simulink model "UAV"  (R2024a)
settings: Solver=FixedStepAuto  StartTime=0  StopTime=inf  MaxStep=0.01  RelTol=1e-4
values from neighbouring files (symbols this model uses):
  actuatorCentres = 0.0    [data.sldd]
  datcom1 : value not decoded    [data.sldd]
  deflectionLimits = -10.0    [data.sldd]
  loggingSampleTime = 1.0    [data.sldd]
  sensorSampleTime = 0.02    [data.sldd]
  vehicle = 1.23    [data.sldd]
undefined symbols (not defined in the file or in its folder): aeroCoeff, aMode, DiscIntNeverNeededParam, Discrete, Earth, HDBK, MIL, Newton, pa28, Raphson, Time, WGS84
libraries: slpidlib x20, simulink_extras x15, simulink x13, arduinolib x8, aerolibasang x5, aerolibactuator x4, aerolibutil x4, aerolibtransform2 x4, sharedtransform x3, ctrlSharedLib x3, aerolibadyn x3, dspstat3 x2
(part 2 of 5)

== system UAV/Arduino/Actuators/Real Actuators/Initialize Function ==
  Aileron Servos : arduinolib/Standard Servo Write  pinNumber=servoPins.aileron.right  ServoIndex=0  blockPlatform=ARDUINO
  Elevator Servo : arduinolib/Standard Servo Write  pinNumber=servoPins.elevator.right  ServoIndex=0  blockPlatform=ARDUINO
  Event Listener : EventListener  DisableCoverage=on  EventName=reset
  Flap Servo : arduinolib/Standard Servo Write  pinNumber=servoPins.flap.right  ServoIndex=0  blockPlatform=ARDUINO
  Rudder Servo : arduinolib/Standard Servo Write  pinNumber=servoPins.rudder  ServoIndex=0  blockPlatform=ARDUINO
  Step : Step  After=180  SampleTime=0
  Step1 : Step  Time=6  After=180  SampleTime=0
  Sum : Sum  Inputs=+-
  wires:
  Sum/1 -> Flap Servo/1, Rudder Servo/1, Elevator Servo/1, Aileron Servos/1
  Step/1 -> Sum/1
  Step1/1 -> Sum/2

== system UAV/Arduino/Flight Control/Model Flight Control/Guidance States/Guidance.ALT_Hold.ALT ==
  Sensors : Inport  OutDataTypeStr=Bus: Sensors
  Demands : Inport  Port=2  OutDataTypeStr=Bus: Demands
  Control Override : Inport  Port=3  OutDataTypeStr=Bus: ControlOverrides
  Action Port : ActionPort
      settings: CopyFcn=Stateflow.SLINSF.SimulinkMan.removeBlockPreDeleteFcn  PreDeleteFcn=Stateflow.SLINSF.SimulinkMan.unsafePredeleteFcn
  Altitude Hold : Subsystem
  Bus Selector : BusSelector  OutputSignals=X_e,phi_theta_psi
  Bus Selector1 : BusSelector  OutputSignals=Altitude
  Bus Selector2 : BusSelector  OutputSignals=Aileron
  Mux : Mux  Inputs=2
  Radians to Degrees : simulink_extras/Transformations/Radians to Degrees
  Rate Limiter : RateLimiter  SampleTimeMode=inherited
  Selector1 : Selector  IndexMode=Zero-based  InputPortWidth=3  IndexOptions=Index vector (dialog)  Indices=[2]  OutputSizes=1
  Selector2 : Selector  IndexMode=Zero-based  InputPortWidth=3  IndexOptions=Index vector (dialog)  Indices=[1]  OutputSizes=1
  Commands : Outport  OutDataTypeStr=single  PortDimensions=2  SampleTime=sensorSampleTime  VectorParamsAs1DForOutWhenUnconnected=off
  wires:
  Mux/1 -> Commands/1
  Altitude Hold/1(Elevator) -> Mux/2
  Selector2/1 -> Radians to Degrees/1
  Sensors/1 -> Bus Selector/1
  Demands/1 -> Bus Selector1/1
  Bus Selector/1 -> Selector1/1  "<X_e>"
  Bus Selector/2 -> Selector2/1  "<phi_theta_psi>"
  Bus Selector1/1 -> Rate Limiter/1  "<Altitude>"
  Rate Limiter/1 -> Altitude Hold/2(Demanded ALT)
  Bus Selector2/1 -> Mux/1  "<Aileron>"
  Control Override/1 -> Bus Selector2/1
  Selector1/1 -> Altitude Hold/1(ALT)
  Radians to Degrees/1 -> Altitude Hold/3(theta)

== system UAV/Arduino/Flight Control/Model Flight Control/Guidance States/Guidance.HDG_ALT_Hold.HDG_ALT ==
  Sensors : Inport  OutDataTypeStr=Bus: Sensors
  Demands : Inport  Port=2  OutDataTypeStr=Bus: Demands
  Action Port : ActionPort
      settings: CopyFcn=Stateflow.SLINSF.SimulinkMan.removeBlockPreDeleteFcn  PreDeleteFcn=Stateflow.SLINSF.SimulinkMan.unsafePredeleteFcn
  Altitude Hold : Subsystem
      settings: UndoDeleteFcn=Stateflow.SLINSF.SimulinkMan.restorePreDeleteFcn  PreDeleteFcn=Stateflow.SLINSF.SimulinkMan.removePreDeleteFcn
  Bus Selector : BusSelector  OutputSignals=phi_theta_psi,X_e
  Bus Selector1 : BusSelector  OutputSignals=Heading,Altitude
  Constant : Constant  Value=360  OutDataTypeStr=single
  Heading Hold : Subsystem
  Mod : Math  Operator=mod  SignedPower=on
  Mux : Mux  Inputs=2
  Radians to Degrees : simulink_extras/Transformations/Radians to Degrees
  Radians to Degrees1 : simulink_extras/Transformations/Radians to Degrees
  Radians to Degrees2 : simulink_extras/Transformations/Radians to Degrees
  Rate Limiter : RateLimiter  SampleTimeMode=inherited
  Rate Limiter1 : RateLimiter  SampleTimeMode=inherited
  Selector : Selector  IndexMode=Zero-based  InputPortWidth=3  IndexOptions=Index vector (dialog)  Indices=[0]  OutputSizes=1
  Selector1 : Selector  IndexMode=Zero-based  InputPortWidth=3  IndexOptions=Index vector (dialog)  Indices=[2]  OutputSizes=1
  Selector2 : Selector  IndexMode=Zero-based  InputPortWidth=3  IndexOptions=Index vector (dialog)  Indices=[1]  OutputSizes=1
  Selector3 : Selector  IndexMode=Zero-based  InputPortWidth=3  IndexOptions=Index vector (dialog)  Indices=[2]  OutputSizes=1
  Commands : Outport  OutDataTypeStr=single  PortDimensions=2  SampleTime=sensorSampleTime  VectorParamsAs1DForOutWhenUnconnected=off
  wires:
  Heading Hold/1(Aileron) -> Mux/1  "Aileron"
  Mux/1 -> Commands/1
  Altitude Hold/1(Elevator) -> Mux/2  "Elevator"
  Selector2/1 -> Radians to Degrees2/1
  Sensors/1 -> Bus Selector/1
  Selector/1 -> Radians to Degrees1/1
  Demands/1 -> Bus Selector1/1
  Bus Selector/2 -> Selector1/1  "<X_e>"
  Bus Selector1/1 -> Rate Limiter/1  "<Heading>"
  Selector3/1 -> Radians to Degrees/1
  Bus Selector/1 -> Selector2/1, Selector/1, Selector3/1  "<phi_theta_psi>"
  Bus Selector1/2 -> Rate Limiter1/1  "<Altitude>"
  Rate Limiter/1 -> Heading Hold/2(Demanded Heading)
  Rate Limiter1/1 -> Altitude Hold/2(ALT Demand)
  Selector1/1 -> Altitude Hold/1(ALT)
  Radians to Degrees/1 -> Mod/1
  Radians to Degrees1/1 -> Heading Hold/3(Current Roll Angle)
  Radians to Degrees2/1 -> Altitude Hold/3(theta)
  Constant/1 -> Mod/2
  Mod/1 -> Heading Hold/1(Current Heading)

== system UAV/Arduino/Flight Control/Model Flight Control/Guidance States/Guidance.HDG_Hold.HDG ==
  Sensors : Inport  OutDataTypeStr=Bus: Sensors
  Demands : Inport  Port=2  OutDataTypeStr=Bus: Demands
  Control Override : Inport  Port=3  OutDataTypeStr=Bus: ControlOverrides
  Action Port : ActionPort
      settings: CopyFcn=Stateflow.SLINSF.SimulinkMan.removeBlockPreDeleteFcn  PreDeleteFcn=Stateflow.SLINSF.SimulinkMan.unsafePredeleteFcn
  Bus Selector : BusSelector  OutputSignals=phi_theta_psi
  Bus Selector1 : BusSelector  OutputSignals=Heading
  Bus Selector2 : BusSelector  OutputSignals=Elevator
  Constant : Constant  Value=360  OutDataTypeStr=single
  Heading Hold : Subsystem
  Mod : Math  Operator=mod  SignedPower=on  OutputSignalType=real
  Mux : Mux  Inputs=2
  Radians to Degrees : simulink_extras/Transformations/Radians to Degrees
  Radians to Degrees1 : simulink_extras/Transformations/Radians to Degrees
  Rate Limiter : RateLimiter  SampleTimeMode=inherited
  Selector : Selector  IndexMode=Zero-based  InputPortWidth=3  IndexOptions=Index vector (dialog)  Indices=[0]  OutputSizes=1
  Selector3 : Selector  IndexMode=Zero-based  InputPortWidth=3  IndexOptions=Index vector (dialog)  Indices=[2]  OutputSizes=1
  Command : Outport  OutDataTypeStr=single  PortDimensions=2  SampleTime=sensorSampleTime  VectorParamsAs1DForOutWhenUnconnected=off
  wires:
  Heading Hold/1(Aileron Command) -> Mux/1  "Aileron"
  Sensors/1 -> Bus Selector/1
  Selector/1 -> Radians to Degrees1/1
  Demands/1 -> Bus Selector1/1
  Bus Selector1/1 -> Rate Limiter/1  "<Heading>"
  Bus Selector/1 -> Selector/1, Selector3/1  "<phi_theta_psi>"
  Rate Limiter/1 -> Heading Hold/2(Demanded Heading)
  Mux/1 -> Command/1
  Control Override/1 -> Bus Selector2/1
  Bus Selector2/1 -> Mux/2  "<Elevator>"
  Selector3/1 -> Radians to Degrees/1
  Radians to Degrees/1 -> Mod/1
  Radians to Degrees1/1 -> Heading Hold/3(Current Roll Angle)
  Mod/1 -> Heading Hold/1(Current Heading)
  Constant/1 -> Mod/2

== system UAV/Arduino/Flight Control/Model Flight Control/HDG_ALT ==
  Sensors : Inport  OutDataTypeStr=Bus: Sensors
  Demands : Inport  Port=2  OutDataTypeStr=Bus: Demands
  Altitude Hold : Subsystem
      settings: UndoDeleteFcn=Stateflow.SLINSF.SimulinkMan.restorePreDeleteFcn  PreDeleteFcn=Stateflow.SLINSF.SimulinkMan.removePreDeleteFcn
  Bus Selector : BusSelector  OutputSignals=phi_theta_psi,X_e
  Bus Selector1 : BusSelector  OutputSignals=Heading,Altitude
  Constant : Constant  Value=360  OutDataTypeStr=single
  Heading Hold : Subsystem
  Mod : Math  Operator=mod  SignedPower=on
  Mux : Mux  Inputs=2
  Radians to Degrees : simulink_extras/Transformations/Radians to Degrees
  Radians to Degrees1 : simulink_extras/Transformations/Radians to Degrees
  Radians to Degrees2 : simulink_extras/Transformations/Radians to Degrees
  Rate Limiter : RateLimiter  SampleTimeMode=inherited
  Rate Limiter1 : RateLimiter  SampleTimeMode=inherited
  Selector : Selector  IndexMode=Zero-based  InputPortWidth=3  IndexOptions=Index vector (dialog)  Indices=[0]  OutputSizes=1
  Selector1 : Selector  IndexMode=Zero-based  InputPortWidth=3  IndexOptions=Index vector (dialog)  Indices=[2]  OutputSizes=1
  Selector2 : Selector  IndexMode=Zero-based  InputPortWidth=3  IndexOptions=Index vector (dialog)  Indices=[1]  OutputSizes=1
  Selector3 : Selector  IndexMode=Zero-based  InputPortWidth=3  IndexOptions=Index vector (dialog)  Indices=[2]  OutputSizes=1
  Commands : Outport  OutDataTypeStr=single  PortDimensions=2  SampleTime=sensorSampleTime  VectorParamsAs1DForOutWhenUnconnected=off
  wires:
  Mod/1 -> Heading Hold/1(Current Heading)
  Constant/1 -> Mod/2
  Radians to Degrees2/1 -> Altitude Hold/3(theta)
  Radians to Degrees1/1 -> Heading Hold/3(Current Roll Angle)
  Radians to Degrees/1 -> Mod/1
  Selector1/1 -> Altitude Hold/1(ALT)
  Rate Limiter1/1 -> Altitude Hold/2(ALT Demand)
  Rate Limiter/1 -> Heading Hold/2(Demanded Heading)
  Bus Selector1/2 -> Rate Limiter1/1  "<Altitude>"
  Bus Selector/1 -> Selector3/1, Selector/1, Selector2/1  "<phi_theta_psi>"
  Selector3/1 -> Radians to Degrees/1
  Bus Selector1/1 -> Rate Limiter/1  "<Heading>"
  Bus Selector/2 -> Selector1/1  "<X_e>"
  Demands/1 -> Bus Selector1/1
  Selector/1 -> Radians to Degrees1/1
  Sensors/1 -> Bus Selector/1
  Selector2/1 -> Radians to Degrees2/1
  Altitude Hold/1(Elevator) -> Mux/2  "Elevator"
  Mux/1 -> Commands/1
  Heading Hold/1(Aileron) -> Mux/1  "Aileron"

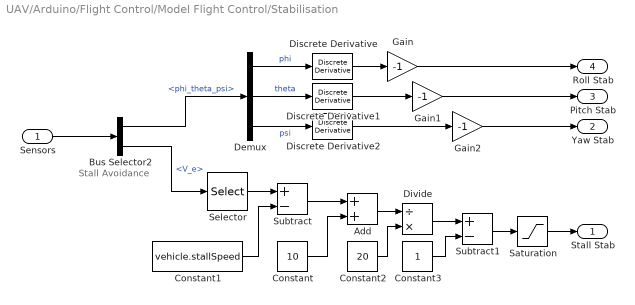
== system UAV/Arduino/Flight Control/Model Flight Control/Stabilisation ==
  note: Stall Avoidance
  Sensors : Inport
  Add : Sum
  Bus Selector2 : BusSelector  OutputSignals=phi_theta_psi,V_e
  Constant : Constant  Value=10  OutDataTypeStr=single
  Constant1 : Constant  Value=vehicle.stallSpeed  OutDataTypeStr=single
  Constant2 : Constant  Value=20  OutDataTypeStr=single
  Constant3 : Constant  OutDataTypeStr=single
  Demux : Demux  Outputs=3
  Discrete Derivative : simulink/Discrete/Discrete Derivative  gainval=1.0  ICPrevScaledInput=0.0  OutMin=[]  OutMax=[]  OutDataType=fixdt(1, 16)  OutScaling=2^-10  DoSatur=off
  Discrete Derivative1 : simulink/Discrete/Discrete Derivative  gainval=1.0  ICPrevScaledInput=0.0  OutMin=[]  OutMax=[]  OutDataType=fixdt(1, 16)  OutScaling=2^-10  DoSatur=off
  Discrete Derivative2 : simulink/Discrete/Discrete Derivative  gainval=1.0  ICPrevScaledInput=0.0  OutMin=[]  OutMax=[]  OutDataType=fixdt(1, 16)  OutScaling=2^-10  DoSatur=off
  Divide : Product  Inputs=/*
  Gain : Gain  Gain=-1
  Gain1 : Gain  Gain=-1
  Gain2 : Gain  Gain=-1
  Saturation : Saturate  UpperLimit=1  LowerLimit=0
  Selector : Selector  IndexMode=Zero-based  InputPortWidth=3  IndexOptions=Index vector (dialog)  Indices=[0]  OutputSizes=1
  Subtract : Sum  Inputs=+-
  Subtract1 : Sum  Inputs=+-
  Stall Stab : Outport  VectorParamsAs1DForOutWhenUnconnected=off
  Yaw Stab : Outport  Port=2  VectorParamsAs1DForOutWhenUnconnected=off
  Pitch Stab : Outport  Port=3  VectorParamsAs1DForOutWhenUnconnected=off
  Roll Stab : Outport  Port=4  VectorParamsAs1DForOutWhenUnconnected=off
  wires:
  Gain2/1 -> Yaw Stab/1
  Bus Selector2/2 -> Selector/1  "<V_e>"
  Discrete Derivative2/1 -> Gain2/1
  Selector/1 -> Subtract/1
  Sensors/1 -> Bus Selector2/1
  Demux/2 -> Discrete Derivative1/1  "theta"
  Demux/1 -> Discrete Derivative/1  "phi"
  Demux/3 -> Discrete Derivative2/1  "psi"
  Discrete Derivative1/1 -> Gain1/1
  Discrete Derivative/1 -> Gain/1
  Bus Selector2/1 -> Demux/1  "<phi_theta_psi>"
  Gain/1 -> Roll Stab/1
  Gain1/1 -> Pitch Stab/1
  Constant1/1 -> Subtract/2
  Saturation/1 -> Stall Stab/1
  Subtract/1 -> Add/1
  Constant/1 -> Add/2
  Add/1 -> Divide/1
  Constant2/1 -> Divide/2
  Divide/1 -> Subtract1/1
  Constant3/1 -> Subtract1/2
  Subtract1/1 -> Saturation/1

== system UAV/Arduino/Flight Control/Real Flight Control/Guidance/Guidance.ALT_Hold.ALT ==
  Sensors : Inport  OutDataTypeStr=Bus: Sensors
  Demands : Inport  Port=2  OutDataTypeStr=Bus: Demands
  Action Port : ActionPort
      settings: CopyFcn=Stateflow.SLINSF.SimulinkMan.removeBlockPreDeleteFcn  PreDeleteFcn=Stateflow.SLINSF.SimulinkMan.unsafePredeleteFcn
  Altitude Hold : Subsystem
  Bus Selector : BusSelector  OutputSignals=Altitude,phi_theta_psi
  Bus Selector1 : BusSelector  OutputSignals=Altitude
  Constant : Constant  Value=0
  Mux : Mux  Inputs=2
  Rate Limiter : RateLimiter  SampleTimeMode=inherited
  Selector2 : Selector  IndexMode=Zero-based  InputPortWidth=3  IndexOptions=Index vector (dialog)  Indices=[1]  OutputSizes=1
  Commands : Outport  VectorParamsAs1DForOutWhenUnconnected=off
  wires:
  Mux/1 -> Commands/1
  Altitude Hold/1(Elevator) -> Mux/2
  Selector2/1 -> Altitude Hold/3(theta)
  Sensors/1 -> Bus Selector/1
  Demands/1 -> Bus Selector1/1
  Bus Selector/1 -> Altitude Hold/1(ALT)  "<Altitude>"
  Bus Selector/2 -> Selector2/1  "<phi_theta_psi>"
  Bus Selector1/1 -> Rate Limiter/1  "<Altitude>"
  Rate Limiter/1 -> Altitude Hold/2(Demanded ALT)
  Constant/1 -> Mux/1

== system UAV/Arduino/Flight Control/Real Flight Control/Guidance/Guidance.HDG_ALT_Hold.HDG_ALT ==
  Sensors : Inport  OutDataTypeStr=Bus: Sensors
  Demands : Inport  Port=2  OutDataTypeStr=Bus: Demands
  Action Port : ActionPort
      settings: CopyFcn=Stateflow.SLINSF.SimulinkMan.removeBlockPreDeleteFcn  PreDeleteFcn=Stateflow.SLINSF.SimulinkMan.unsafePredeleteFcn
  Altitude Hold : Subsystem
      settings: UndoDeleteFcn=Stateflow.SLINSF.SimulinkMan.restorePreDeleteFcn  PreDeleteFcn=Stateflow.SLINSF.SimulinkMan.removePreDeleteFcn
  Bus Selector : BusSelector  OutputSignals=Heading,phi_theta_psi,Altitude
  Bus Selector1 : BusSelector  OutputSignals=Heading,Altitude
  Heading Hold : Subsystem
  Mux : Mux  Inputs=2
  Rate Limiter : RateLimiter  SampleTimeMode=inherited
  Rate Limiter1 : RateLimiter  SampleTimeMode=inherited
  Selector : Selector  IndexMode=Zero-based  InputPortWidth=3  IndexOptions=Index vector (dialog)  Indices=[0]  OutputSizes=1
  Selector2 : Selector  IndexMode=Zero-based  InputPortWidth=3  IndexOptions=Index vector (dialog)  Indices=[1]  OutputSizes=1
  Commands : Outport  VectorParamsAs1DForOutWhenUnconnected=off
  wires:
  Heading Hold/1(Aileron) -> Mux/1  "Aileron"
  Mux/1 -> Commands/1
  Altitude Hold/1(Elevator) -> Mux/2  "Elevator"
  Selector2/1 -> Altitude Hold/3(theta)
  Sensors/1 -> Bus Selector/1
  Selector/1 -> Heading Hold/3(Current Roll Angle)
  Demands/1 -> Bus Selector1/1
  Bus Selector/3 -> Altitude Hold/1(ALT)  "<Altitude>"
  Bus Selector1/1 -> Rate Limiter/1  "<Heading>"
  Bus Selector/1 -> Heading Hold/1(Current Heading)  "<Heading>"
  Bus Selector/2 -> Selector2/1, Selector/1  "<phi_theta_psi>"
  Bus Selector1/2 -> Rate Limiter1/1  "<Altitude>"
  Rate Limiter/1 -> Heading Hold/2(Demanded Heading)
  Rate Limiter1/1 -> Altitude Hold/2(ALT Demand)

== system UAV/Arduino/Flight Control/Real Flight Control/Guidance/Guidance.HDG_Hold.HDG ==
  Sensors : Inport  OutDataTypeStr=Bus: Sensors
  Demands : Inport  Port=2  OutDataTypeStr=Bus: Demands
  Action Port : ActionPort
      settings: CopyFcn=Stateflow.SLINSF.SimulinkMan.removeBlockPreDeleteFcn  PreDeleteFcn=Stateflow.SLINSF.SimulinkMan.unsafePredeleteFcn
  Bus Selector : BusSelector  OutputSignals=Heading,phi_theta_psi
  Bus Selector1 : BusSelector  OutputSignals=Heading
  Constant : Constant  Value=0
  Heading Hold : Subsystem
  Mux : Mux  Inputs=2
  Rate Limiter : RateLimiter  SampleTimeMode=inherited
  Selector : Selector  IndexMode=Zero-based  InputPortWidth=3  IndexOptions=Index vector (dialog)  Indices=[0]  OutputSizes=1
  Command : Outport  VectorParamsAs1DForOutWhenUnconnected=off
  wires:
  Heading Hold/1(Aileron Command) -> Mux/1  "Aileron"
  Sensors/1 -> Bus Selector/1
  Selector/1 -> Heading Hold/3(Current Roll Angle)
  Demands/1 -> Bus Selector1/1
  Bus Selector1/1 -> Rate Limiter/1  "<Heading>"
  Bus Selector/1 -> Heading Hold/1(Current Heading)  "<Heading>"
  Bus Selector/2 -> Selector/1  "<phi_theta_psi>"
  Rate Limiter/1 -> Heading Hold/2(Demanded Heading)
  Mux/1 -> Command/1
  Constant/1 -> Mux/2

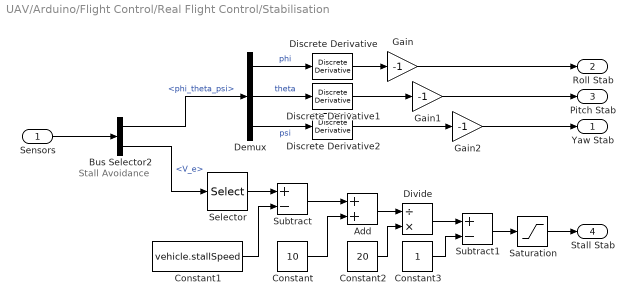
== system UAV/Arduino/Flight Control/Real Flight Control/Stabilisation ==
  note: Stall Avoidance
  Sensors : Inport
  Add : Sum
  Bus Selector2 : BusSelector  OutputSignals=phi_theta_psi,V_e
  Constant : Constant  Value=10  OutDataTypeStr=single
  Constant1 : Constant  Value=vehicle.stallSpeed  OutDataTypeStr=single
  Constant2 : Constant  Value=20  OutDataTypeStr=single
  Constant3 : Constant  OutDataTypeStr=single
  Demux : Demux  Outputs=3
  Discrete Derivative : simulink/Discrete/Discrete Derivative  gainval=1.0  ICPrevScaledInput=0.0  OutMin=[]  OutMax=[]  OutDataType=fixdt(1, 16)  OutScaling=2^-10  DoSatur=off
  Discrete Derivative1 : simulink/Discrete/Discrete Derivative  gainval=1.0  ICPrevScaledInput=0.0  OutMin=[]  OutMax=[]  OutDataType=fixdt(1, 16)  OutScaling=2^-10  DoSatur=off
  Discrete Derivative2 : simulink/Discrete/Discrete Derivative  gainval=1.0  ICPrevScaledInput=0.0  OutMin=[]  OutMax=[]  OutDataType=fixdt(1, 16)  OutScaling=2^-10  DoSatur=off
  Divide : Product  Inputs=/*
  Gain : Gain  Gain=-1
  Gain1 : Gain  Gain=-1
  Gain2 : Gain  Gain=-1
  Saturation : Saturate  UpperLimit=1  LowerLimit=0
  Selector : Selector  IndexMode=Zero-based  InputPortWidth=3  IndexOptions=Index vector (dialog)  Indices=[0]  OutputSizes=1
  Subtract : Sum  Inputs=+-
  Subtract1 : Sum  Inputs=+-
  Yaw Stab : Outport  VectorParamsAs1DForOutWhenUnconnected=off
  Roll Stab : Outport  Port=2  VectorParamsAs1DForOutWhenUnconnected=off
  Pitch Stab : Outport  Port=3  VectorParamsAs1DForOutWhenUnconnected=off
  Stall Stab : Outport  Port=4  VectorParamsAs1DForOutWhenUnconnected=off
  wires:
  Gain2/1 -> Yaw Stab/1
  Bus Selector2/2 -> Selector/1  "<V_e>"
  Discrete Derivative2/1 -> Gain2/1
  Selector/1 -> Subtract/1
  Sensors/1 -> Bus Selector2/1
  Demux/2 -> Discrete Derivative1/1  "theta"
  Demux/1 -> Discrete Derivative/1  "phi"
  Demux/3 -> Discrete Derivative2/1  "psi"
  Discrete Derivative1/1 -> Gain1/1
  Discrete Derivative/1 -> Gain/1
  Bus Selector2/1 -> Demux/1  "<phi_theta_psi>"
  Gain/1 -> Roll Stab/1
  Gain1/1 -> Pitch Stab/1
  Constant1/1 -> Subtract/2
  Saturation/1 -> Stall Stab/1
  Subtract/1 -> Add/1
  Constant/1 -> Add/2
  Add/1 -> Divide/1
  Constant2/1 -> Divide/2
  Divide/1 -> Subtract1/1
  Constant3/1 -> Subtract1/2
  Subtract1/1 -> Saturation/1

== system UAV/Arduino/Sensors/Model Sensors/3 NaN check ==
  In2 : Inport
  Relational Operator1 : RelationalOperator  Operator=isNaN  OutDataTypeStr=boolean  RndMeth=Simplest  InputSameDT=off
  Switch1 : Switch  Criteria=u2 ~= 0  SaturateOnIntegerOverflow=off  InputSameDT=off
  Unit Delay5 : UnitDelay  InitialCondition=[0; 0; 0]  SampleTime=-1  HasFrameUpgradeWarning=on
  Out1 : Outport  VectorParamsAs1DForOutWhenUnconnected=off
  wires:
  Relational Operator1/1 -> Switch1/2
  Unit Delay5/1 -> Switch1/1
  Switch1/1 -> Unit Delay5/1, Out1/1
  In2/1 -> Relational Operator1/1, Switch1/3

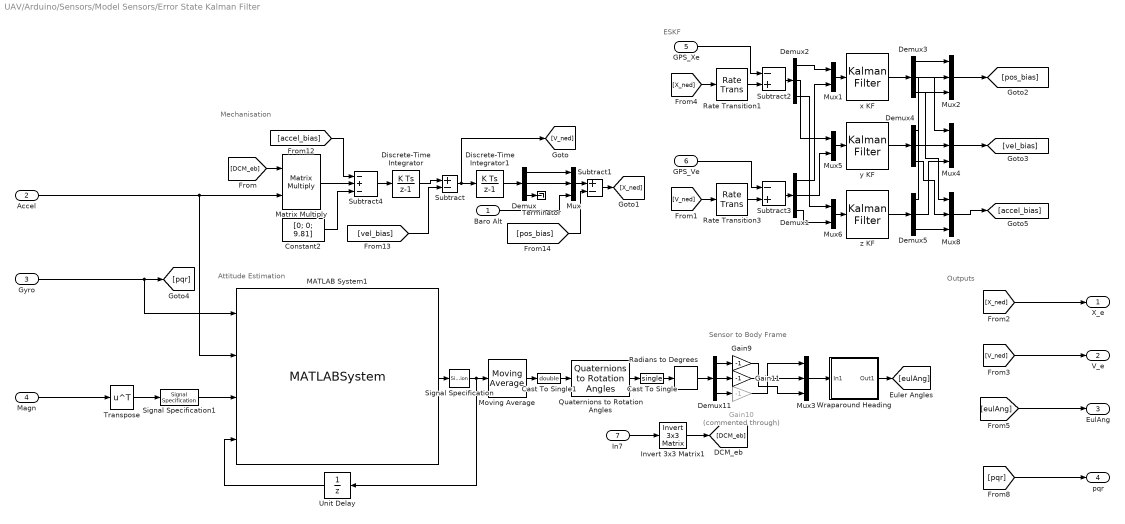
== system UAV/Arduino/Sensors/Model Sensors/Error State Kalman Filter ==
  note: Attitude Estimation
  note: Mechanisation
  note: ESKF
  note: Outputs
  note: Sensor to Body Frame
  Baro Alt : Inport
  Accel : Inport  Port=2
  Gyro : Inport  Port=3
  Magn : Inport  Port=4
  GPS_Xe : Inport  Port=5
  GPS_Ve : Inport  Port=6
  In7 : Inport  Port=7
  Cast To Single : DataTypeConversion  OutDataTypeStr=single  RndMeth=Simplest  SaturateOnIntegerOverflow=off
  Cast To Single1 : DataTypeConversion  OutDataTypeStr=double  RndMeth=Simplest  SaturateOnIntegerOverflow=off
  Constant2 : Constant  Value=[0; 0; 9.81]  VectorParams1D=off  OutDataTypeStr=single
  Demux{,1..5,11} (7 alike) : Demux  Outputs=3
  Discrete-Time Integrator : DiscreteIntegrator  gainval=1  SampleTime=-1  ICPrevOutput=DiscIntNeverNeededParam  ICPrevScaledInput=DiscIntNeverNeededParam
  Discrete-Time Integrator1 : DiscreteIntegrator  gainval=1  SampleTime=-1  OutDataTypeStr=single  ICPrevOutput=DiscIntNeverNeededParam  ICPrevScaledInput=DiscIntNeverNeededParam
  Gain10 : Gain  Commented=through  Gain=-1
  Gain11 : Gain  Gain=-1
  Gain9 : Gain  Gain=-1
  Invert 3x3 Matrix1 : aerolibutil/Invert  3x3 Matrix
  MATLAB System1 : MATLABSystem  System=MadgwickAHRSFilter  SamplePeriod=sensorSampleTime  Beta=5  SimulateUsing=Code generation
      mask Type: MadgwickAHRSFilter
      mask Display:
      | disp('MadgwickAHRSFilter');
      | port_label('input',1,'Gyroscope');
      | port_label('input',2,'Accelerometer');
      | port_label('input',3,'Magnetometer');
      | port_label('input',4,'q');
      | port_label('output',1,'quat');
  Matrix Multiply : Product  Multiplication=Matrix(*)  OutDataTypeStr=single  RndMeth=Simplest
  Moving Average : dspstat3/Moving Average  Method=Exponential weighting  ForgettingFactorPort=off  SpecifyWindowLength=on  WindowLength=4  OverlapLength=3  AllowArbitraryInputLength=off  ForgettingFactor=0.12  SimulateUsing=Code generation
  Mux{,2..4,8} (5 alike) : Mux  Inputs=3
  Mux1 : Mux  Inputs=2
  Mux5 : Mux  Inputs=2
  Mux6 : Mux  Inputs=2
  Quaternions to Rotation Angles : sharedtransform/Quaternions to Rotation Angles  rotationOrder=ZYX  aMode=aMode
  Radians to Degrees : simulink_extras/Transformations/Radians to Degrees
  Rate Transition1 : RateTransition  OutPortSampleTime=1
  Rate Transition3 : RateTransition  OutPortSampleTime=1
  Signal Specification : SignalSpecification  Dimensions=[1 4]
  Signal Specification1 : SignalSpecification  OutDataTypeStr=single  Dimensions=[1 3]
  Subtract : Sum  Inputs=+-
  Subtract1 : Sum  Inputs=+-
  Subtract2 : Sum  Inputs=-+  OutDataTypeStr=single  AccumDataTypeStr=single  RndMeth=Simplest
  Subtract3 : Sum  Inputs=-+  OutDataTypeStr=single  AccumDataTypeStr=single  RndMeth=Simplest
  Subtract4 : Sum  Inputs=-+-  AccumDataTypeStr=single
  Terminator : Terminator
  Transpose : Math  Operator=transpose  SignedPower=on
  Unit Delay : UnitDelay  InitialCondition=[1 0 0 0]  SampleTime=sensorSampleTime  HasFrameUpgradeWarning=on
  Wraparound Heading : Subsystem
  x KF : ctrlSharedLib/Kalman Filter  TimeDomain=Discrete-Time  UseCurrentEstimator=off  ModelSource=Individual A, B, C, D matrices  ModelSourceVariable=ss(0.95,1,1,0,1)  A=[1 0.2 0.02; 0 1 0.2; 0 0 1]  B=0  C=[1 0 0; 0 1 0]  D=0  NumberOfStates=3  NumberOfInputs=1  NumberOfOutputs=3  InitialEstimateSource=Dialog  X0=[0;0;0]  P0=10  UseK=off  UseGH=off  NumberOfProcessNoiseInputs=1  G=1  TimeInvariantG=on  H=0  TimeInvariantH=on  Q=0.5  TimeInvariantQ=on  R=0.1  TimeInvariantR=on  N=0  TimeInvariantN=on  AddInputPort=off  AddEnablePort=off  OutputEstimatedY=off  OutputP=off  Ts=1
  y KF : ctrlSharedLib/Kalman Filter  TimeDomain=Discrete-Time  UseCurrentEstimator=off  ModelSource=Individual A, B, C, D matrices  ModelSourceVariable=ss(0.95,1,1,0,1)  A=[1 1 0.5; 0 1 1; 0 0 1]  B=0  C=[1 0 0; 0 1 0]  D=0  NumberOfStates=3  NumberOfInputs=1  NumberOfOutputs=3  InitialEstimateSource=Dialog  X0=[0;0;0]  P0=10  UseK=off  UseGH=off  NumberOfProcessNoiseInputs=1  G=1  TimeInvariantG=on  H=0  TimeInvariantH=on  Q=0.5  TimeInvariantQ=on  R=0.1  TimeInvariantR=on  N=0  TimeInvariantN=on  AddInputPort=off  AddEnablePort=off  OutputEstimatedY=off  OutputP=off  Ts=1
  z KF : ctrlSharedLib/Kalman Filter  TimeDomain=Discrete-Time  UseCurrentEstimator=off  ModelSource=Individual A, B, C, D matrices  ModelSourceVariable=ss(0.95,1,1,0,1)  A=[1 1 0.5; 0 1 1; 0 0 1]  B=0  C=[1 0 0; 0 1 0]  D=0  NumberOfStates=3  NumberOfInputs=1  NumberOfOutputs=3  InitialEstimateSource=Dialog  X0=[0;0;0]  P0=10  UseK=off  UseGH=off  NumberOfProcessNoiseInputs=1  G=1  TimeInvariantG=on  H=0  TimeInvariantH=on  Q=0.5  TimeInvariantQ=on  R=0.1  TimeInvariantR=on  N=0  TimeInvariantN=on  AddInputPort=off  AddEnablePort=off  OutputEstimatedY=off  OutputP=off  Ts=1
  X_e : Outport  VectorParamsAs1DForOutWhenUnconnected=off
  V_e : Outport  Port=2  VectorParamsAs1DForOutWhenUnconnected=off
  EulAng : Outport  Port=3  VectorParamsAs1DForOutWhenUnconnected=off
  pqr : Outport  Port=4  VectorParamsAs1DForOutWhenUnconnected=off
  wires:
  Accel/1 -> MATLAB System1/2, Matrix Multiply/2
  [DCM_eb] -> Matrix Multiply/1
  Matrix Multiply/1 -> Subtract4/2
  Discrete-Time Integrator1/1 -> Demux/1
  Demux/1 -> Mux/1
  Demux/2 -> Mux/2
  Baro Alt/1 -> Mux/3
  Demux/3 -> Terminator/1
  GPS_Xe/1 -> Subtract2/1
  GPS_Ve/1 -> Subtract3/1
  Subtract4/1 -> Discrete-Time Integrator/1
  Constant2/1 -> Subtract4/3
  Mux/1 -> Subtract1/1
  Discrete-Time Integrator/1 -> Subtract/1
  [X_ned] -> X_e/1
  [V_ned] -> V_e/1
  Unit Delay/1 -> MATLAB System1/4
  Demux11/3 -> Gain10/1
  Quaternions to Rotation Angles/1 -> Cast To Single/1
  Gain9/1 -> Mux3/3
  Gain11/1 -> Mux3/2
  Demux11/1 -> Gain9/1
  Wraparound Heading/1(Out1) -> [eulAng]
  MATLAB System1/1 -> Signal Specification/1
  Gain10/1 -> Mux3/1
  Demux11/2 -> Gain11/1
  Radians to Degrees/1 -> Demux11/1
  Mux3/1 -> Wraparound Heading/1(In1)
  Invert 3x3 Matrix1/1 -> [DCM_eb]
  In7/1 -> Invert 3x3 Matrix1/1
  Gyro/1 -> MATLAB System1/1, [pqr]
  Transpose/1 -> Signal Specification1/1
  [pqr] -> pqr/1
  Magn/1 -> Transpose/1
  [eulAng] -> EulAng/1
  Signal Specification/1 -> Moving Average/1, Unit Delay/1
  Signal Specification1/1 -> MATLAB System1/3
  Subtract/1 -> Discrete-Time Integrator1/1, [V_ned]
  [V_ned] -> Rate Transition3/1
  [X_ned] -> Rate Transition1/1
  Mux1/1 -> x KF/1
  Mux5/1 -> y KF/1
  Mux6/1 -> z KF/1
  Demux2/1 -> Mux1/1
  Demux1/1 -> Mux1/2
  Demux2/2 -> Mux5/1
  Demux1/2 -> Mux5/2
  Demux2/3 -> Mux6/1
  Demux1/3 -> Mux6/2
  x KF/1 -> Demux3/1
  y KF/1 -> Demux4/1
  z KF/1 -> Demux5/1
  Demux3/1 -> Mux2/1
  Demux4/1 -> Mux2/2
  Demux5/1 -> Mux2/3
  Demux3/2 -> Mux4/1
  Demux4/2 -> Mux4/2
  Demux5/2 -> Mux4/3
  Demux3/3 -> Mux8/1
  Demux4/3 -> Mux8/2
  Demux5/3 -> Mux8/3
  [accel_bias] -> Subtract4/1
  [vel_bias] -> Subtract/2
  Subtract1/1 -> [X_ned]
  [pos_bias] -> Subtract1/2
  Subtract2/1 -> Demux2/1
  Subtract3/1 -> Demux1/1
  Rate Transition1/1 -> Subtract2/2
  Rate Transition3/1 -> Subtract3/2
  Cast To Single/1 -> Radians to Degrees/1
  Moving Average/1 -> Cast To Single1/1
  Mux2/1 -> [pos_bias]
  Mux4/1 -> [vel_bias]
  Mux8/1 -> [accel_bias]
  Cast To Single1/1 -> Quaternions to Rotation Angles/1

== system UAV/Arduino/Sensors/Real Sensors/3 NaN check1 ==
  In2 : Inport
  Relational Operator1 : RelationalOperator  Operator=isNaN  OutDataTypeStr=boolean  RndMeth=Simplest  InputSameDT=off
  Switch1 : Switch  Criteria=u2 ~= 0  SaturateOnIntegerOverflow=off  InputSameDT=off
  Unit Delay5 : UnitDelay  InitialCondition=[0; 0; 0]  SampleTime=-1  HasFrameUpgradeWarning=on
  Out1 : Outport  VectorParamsAs1DForOutWhenUnconnected=off
  wires:
  Relational Operator1/1 -> Switch1/2
  Unit Delay5/1 -> Switch1/1
  Switch1/1 -> Unit Delay5/1, Out1/1
  In2/1 -> Relational Operator1/1, Switch1/3

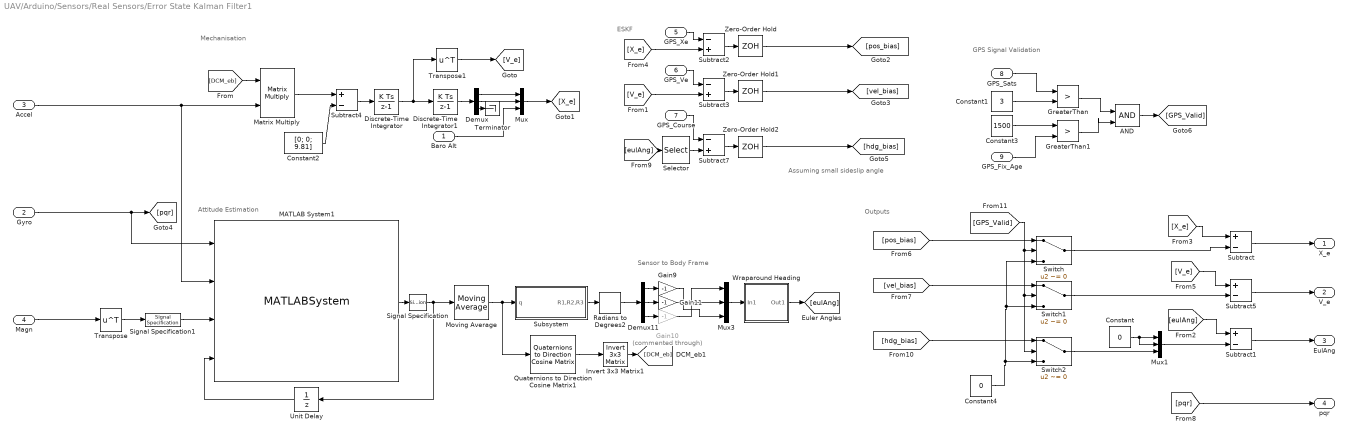
== system UAV/Arduino/Sensors/Real Sensors/Error State Kalman Filter1 ==
  note: GPS Signal Validation
  note: Assuming small sideslip angle
  note: Attitude Estimation
  note: Mechanisation
  note: ESKF
  note: Outputs
  note: Sensor to Body Frame
  Baro Alt : Inport
  Gyro : Inport  Port=2
  Accel : Inport  Port=3
  Magn : Inport  Port=4
  GPS_Xe : Inport  Port=5  OutDataTypeStr=single
  GPS_Ve : Inport  Port=6  OutDataTypeStr=single
  GPS_Course : Inport  Port=7  OutDataTypeStr=single
  GPS_Sats : Inport  Port=8
  GPS_Fix_Age : Inport  Port=9
  AND : Logic  IconShape=distinctive  AllPortsSameDT=off  OutDataTypeStr=boolean
  Constant : Constant  Value=0
  Constant1 : Constant  Value=3
  Constant2 : Constant  Value=[0; 0; 9.81]  VectorParams1D=off  OutDataTypeStr=single
  Constant3 : Constant  Value=1500
  Constant4 : Constant  Value=0
  Demux : Demux  Outputs=3
  Demux11 : Demux  Outputs=3
  Discrete-Time Integrator : DiscreteIntegrator  SampleTime=-1  RndMeth=Simplest  LimitOutput=on  UpperSaturationLimit=500  LowerSaturationLimit=-500  ICPrevOutput=DiscIntNeverNeededParam  ICPrevScaledInput=DiscIntNeverNeededParam
  Discrete-Time Integrator1 : DiscreteIntegrator  SampleTime=-1  RndMeth=Simplest  LimitOutput=on  UpperSaturationLimit=500  LowerSaturationLimit=-500  ICPrevOutput=DiscIntNeverNeededParam  ICPrevScaledInput=DiscIntNeverNeededParam
  Gain10 : Gain  Commented=through  Gain=-1
  Gain11 : Gain  Gain=-1
  Gain9 : Gain  Gain=-1
  GreaterThan : RelationalOperator  Operator=>  OutDataTypeStr=boolean  RndMeth=Simplest  InputSameDT=off
  GreaterThan1 : RelationalOperator  Operator=>  OutDataTypeStr=boolean  RndMeth=Simplest  InputSameDT=off
  Invert 3x3 Matrix1 : aerolibutil/Invert  3x3 Matrix
  MATLAB System1 : MATLABSystem  System=MadgwickAHRSFilter  SamplePeriod=sensorSampleTime  Beta=5  SimulateUsing=Code generation
      mask Type: MadgwickAHRSFilter
      mask Display:
      | disp('MadgwickAHRSFilter');
      | port_label('input',1,'Gyroscope');
      | port_label('input',2,'Accelerometer');
      | port_label('input',3,'Magnetometer');
      | port_label('input',4,'q');
      | port_label('output',1,'quat');
  Matrix Multiply : Product  Multiplication=Matrix(*)
  Moving Average : dspstat3/Moving Average  Method=Exponential weighting  ForgettingFactorPort=off  SpecifyWindowLength=off  WindowLength=4  OverlapLength=3  AllowArbitraryInputLength=off  ForgettingFactor=0.9  SimulateUsing=Code generation
  Mux : Mux  Inputs=3
  Mux1 : Mux  Inputs=3
  Mux3 : Mux  Inputs=3
  Quaternions to Direction Cosine Matrix1 : sharedtransform/Quaternions to  Direction Cosine Matrix  aMode=aMode
  Radians to Degrees2 : simulink_extras/Transformations/Radians to Degrees
  Selector : Selector  IndexMode=Zero-based  InputPortWidth=3  IndexOptions=Index vector (dialog)  Indices=[2]  OutputSizes=1
  Signal Specification : SignalSpecification  OutDataTypeStr=single  Dimensions=[1 4]
  Signal Specification1 : SignalSpecification  OutDataTypeStr=single  Dimensions=[1 3]
  Subsystem : Subsystem
  Subtract : Sum  Inputs=+-
  Subtract1 : Sum  Inputs=+-
  Subtract2 : Sum  Inputs=-+  AccumDataTypeStr=single
  Subtract3 : Sum  Inputs=-+  AccumDataTypeStr=single
  Subtract4 : Sum  Inputs=+-  AccumDataTypeStr=single
  Subtract5 : Sum  Inputs=+-
  Subtract7 : Sum  Inputs=-+  AccumDataTypeStr=single
  Switch : Switch  Criteria=u2 ~= 0  SaturateOnIntegerOverflow=off  InputSameDT=off
  Switch1 : Switch  Criteria=u2 ~= 0  SaturateOnIntegerOverflow=off  InputSameDT=off
  Switch2 : Switch  Criteria=u2 ~= 0  SaturateOnIntegerOverflow=off  InputSameDT=off
  Terminator : Terminator
  Transpose : Math  Operator=transpose  SignedPower=on
  Transpose1 : Math  Operator=transpose  SignedPower=on
  Unit Delay : UnitDelay  InitialCondition=[1 0 0 0]  SampleTime=sensorSampleTime  HasFrameUpgradeWarning=on
  Wraparound Heading : Subsystem
  Zero-Order Hold : ZeroOrderHold
  Zero-Order Hold1 : ZeroOrderHold
  Zero-Order Hold2 : ZeroOrderHold
  X_e : Outport  VectorParamsAs1DForOutWhenUnconnected=off
  V_e : Outport  Port=2  VectorParamsAs1DForOutWhenUnconnected=off
  EulAng : Outport  Port=3  VectorParamsAs1DForOutWhenUnconnected=off
  pqr : Outport  Port=4  VectorParamsAs1DForOutWhenUnconnected=off
  wires:
  Accel/1 -> MATLAB System1/2, Matrix Multiply/2
  [DCM_eb] -> Matrix Multiply/1
  Matrix Multiply/1 -> Subtract4/1
  Discrete-Time Integrator1/1 -> Demux/1
  Demux/1 -> Mux/1
  Demux/2 -> Mux/2
  Baro Alt/1 -> Mux/3
  Demux/3 -> Terminator/1
  GPS_Xe/1 -> Subtract2/1
  GPS_Ve/1 -> Subtract3/1
  Subtract2/1 -> Zero-Order Hold/1
  Subtract3/1 -> Zero-Order Hold1/1
  Subtract4/1 -> Discrete-Time Integrator/1
  Constant2/1 -> Subtract4/2
  Mux/1 -> [X_e]
  Discrete-Time Integrator/1 -> Transpose1/1, Discrete-Time Integrator1/1
  [eulAng] -> Subtract1/1
  [X_e] -> Subtract/1
  Subtract/1 -> X_e/1
  [pos_bias] -> Switch/1
  [V_e] -> Subtract5/1
  Subtract5/1 -> V_e/1
  [vel_bias] -> Switch1/1
  Unit Delay/1 -> MATLAB System1/4
  Demux11/3 -> Gain10/1
  Subsystem/1(R1,R2,R3) -> Radians to Degrees2/1
  Gain9/1 -> Mux3/3
  Gain11/1 -> Mux3/2
  Demux11/1 -> Gain9/1
  Wraparound Heading/1(Out1) -> [eulAng]
  MATLAB System1/1 -> Signal Specification/1
  Gain10/1 -> Mux3/1
  Demux11/2 -> Gain11/1
  Signal Specification/1 -> Moving Average/1, Unit Delay/1
  Radians to Degrees2/1 -> Demux11/1
  Mux3/1 -> Wraparound Heading/1(In1)
  Invert 3x3 Matrix1/1 -> [DCM_eb]
  Quaternions to Direction Cosine Matrix1/1 -> Invert 3x3 Matrix1/1
  Gyro/1 -> MATLAB System1/1, [pqr]
  Transpose/1 -> Signal Specification1/1
  [pqr] -> pqr/1
  Magn/1 -> Transpose/1
  Subtract7/1 -> Zero-Order Hold2/1
  GPS_Course/1 -> Subtract7/1
  Subtract1/1 -> EulAng/1
  Mux1/1 -> Subtract1/2
  [hdg_bias] -> Switch2/1
  Constant/1 -> Mux1/2, Mux1/1
  Selector/1 -> Subtract7/2
  GreaterThan1/1 -> AND/2
  GreaterThan/1 -> AND/1
  AND/1 -> [GPS_Valid]
  GPS_Sats/1 -> GreaterThan/1
  GPS_Fix_Age/1 -> GreaterThan1/2
  Constant1/1 -> GreaterThan/2
  Constant3/1 -> GreaterThan1/1
  [GPS_Valid] -> Switch2/2, Switch1/2, Switch/2
  Switch2/1 -> Mux1/3
  Switch1/1 -> Subtract5/2
  Switch/1 -> Subtract/2
  Constant4/1 -> Switch/3, Switch1/3, Switch2/3
  Signal Specification1/1 -> MATLAB System1/3
  Transpose1/1 -> [V_e]
  Zero-Order Hold/1 -> [pos_bias]
  Zero-Order Hold1/1 -> [vel_bias]
  [V_e] -> Subtract3/2
  [X_e] -> Subtract2/2
  [eulAng] -> Selector/1
  Zero-Order Hold2/1 -> [hdg_bias]
  Moving Average/1 -> Subsystem/1(q), Quaternions to Direction Cosine Matrix1/1

== system UAV/Arduino/Sensors/Real Sensors/GPS Init1 ==
  note: GPS Signal Validation
  GPS_LL : Inport
  GPS_Alt : Inport  Port=2
  GPS_Sats : Inport  Port=3
  GPS_Fix_Age : Inport  Port=4
  AND : Logic  IconShape=distinctive  AllPortsSameDT=off  OutDataTypeStr=boolean
  Constant1 : Constant  Value=3  OutDataTypeStr=single
  Constant3 : Constant  Value=1500  OutDataTypeStr=single
  Data Store Memory : DataStoreMemory  DataStoreName=GPS_init  ReadBeforeWriteMsg=warning  WriteAfterWriteMsg=warning  WriteAfterReadMsg=warning  InitialValue=true  ShowAdditionalParam=off  OutDataTypeStr=boolean
  Data Store Read : DataStoreRead  DataStoreName=GPS_init  DataStoreElements=GPS_init  IndexOptions=Index vector (dialog)  Indices=1  OutputSizes=1
  GreaterThan : RelationalOperator  Operator=>  OutDataTypeStr=boolean  RndMeth=Simplest  InputSameDT=off
  GreaterThan1 : RelationalOperator  Operator=>  OutDataTypeStr=boolean  RndMeth=Simplest  InputSameDT=off
  If : If  NumInputs=2  IfExpression=(u1 ~= 0) & (u2 ~=2)  ShowElse=off
  If Action Subsystem : Subsystem  TreatAsAtomicUnit=on
  Initialize Function : Subsystem  TreatAsAtomicUnit=on
  wires:
  GreaterThan/1 -> AND/1
  Constant3/1 -> GreaterThan1/1
  GPS_Fix_Age/1 -> GreaterThan1/2
  GreaterThan1/1 -> AND/2
  Constant1/1 -> GreaterThan/2
  GPS_Sats/1 -> GreaterThan/1
  AND/1 -> If/2
  Data Store Read/1 -> If/1
  If/1 -> If Action Subsystem/Action
  GPS_Alt/1 -> If Action Subsystem/2(GPS_Alt)
  GPS_LL/1 -> If Action Subsystem/1(GPS_LL)

== system UAV/Arduino/Sensors/Real Sensors/LLA to Flat Earth1 ==
  mu l : Inport  Unit=deg
  h : Inport  Port=2  Unit=m
  ground height : Inport  Port=3  Unit=m
  Ref LL : Inport  Port=4
  Disallow CGS : UnitConfiguration  UnitSystemsStr=English,SI,SI (extended)  AllowAllUnitSystems=off
  LatLong wrap : Subsystem  AncestorBlock=aerolibtransform2sys/LatLong wrap
      mask init:
      | aeroicon('aeroblk')
      mask Display:
      | port_label('input',1,'[\mu l]','texmode','on')
      | port_label('output',1,'[\mu l]_{wrap}','texmode','on')
  LatLong wrap LL0 : Subsystem  AncestorBlock=aerolibtransform2sys/LatLong wrap
      mask init:
      | aeroicon('aeroblk')
      mask Display:
      | port_label('input',1,'[\mu l]','texmode','on')
      | port_label('output',1,'[\mu l]_{wrap}','texmode','on')
  Mux : Mux  Inputs=3
  Subsystem1 : Subsystem
  Sum : Sum  Inputs=++|
  Sum1 : Sum  Inputs=-+|
  Ze2height : UnaryMinus
  initial_latg : Selector  IndexMode=Zero-based  InputPortWidth=2  IndexOptions=Index vector (dialog)  Indices=[1]  OutputSizes=1
  pos_rad : aerolibtransform2/LLA to Flat Earth/pos_rad  SystemSampleTime=-1  VariantActivationTime=update diagram  AllowFlexibleInterface=on  Latency=0  AutoFrameSizeCalculation=off
  Xe : Outport  Unit=m  VectorParamsAs1DForOutWhenUnconnected=off
  wires:
  LatLong wrap LL0/1(Lat/Long wrapped) -> initial_latg/1, Sum1/1
  pos_rad/1 -> Subsystem1/1(pos_rad)
  Sum1/1 -> LatLong wrap/1(LatLong)
  Subsystem1/2(Py) -> Mux/2
  Subsystem1/1(Px) -> Mux/1
  Ze2height/1 -> Mux/3  "Pz"
  Mux/1 -> Xe/1
  initial_latg/1 -> Subsystem1/2(mu)
  h/1 -> Sum/1
  Ref LL/1 -> LatLong wrap LL0/1(LatLong)
  ground height/1 -> Sum/2
  mu l/1 -> Sum1/2
  LatLong wrap/1(Lat/Long wrapped) -> pos_rad/1
  Sum/1 -> Ze2height/1  "alt"

== system UAV/Arduino/Sensors/Real Sensors/Real Sensors ==
  MATLAB System : MATLABSystem  System=BMP085  Reference_Pressure=101200  SimulateUsing=Code generation
      mask Type: BMP085
      mask Display:
      | disp('BMP085');
      | port_label('output',1,'press');
      | port_label('output',2,'temp');
      | port_label('output',3,'alt');
  MATLAB System1 : MATLABSystem  System=L3GD20  SimulateUsing=Code generation
      mask Type: L3GD20
      mask Display:
      | disp('L3GD20');
      | port_label('output',1,'rot');
  MATLAB System2 : MATLABSystem  System=LSM303  SimulateUsing=Code generation
      mask Type: LSM303
      mask Display:
      | disp('LSM303');
      | port_label('output',1,'accel');
      | port_label('output',2,'mag');
  MATLAB System3 : MATLABSystem  System=TinyGPS  SimulateUsing=Code generation
      mask Type: TinyGPS
      mask Display:
      | disp('TinyGPS');
      | port_label('output',1,'lat');
      | port_label('output',2,'lon');
      | port_label('output',3,'speed');
      | port_label('output',4,'course');
      | port_label('output',5,'alt');
      | port_label('output',6,'sats');
      | port_label('output',7,'age');
  Terminator : Terminator
  Terminator1 : Terminator
  Baro_Alt : Outport  VectorParamsAs1DForOutWhenUnconnected=off
  RotVel : Outport  Port=2  VectorParamsAs1DForOutWhenUnconnected=off
  LinAccel : Outport  Port=3  VectorParamsAs1DForOutWhenUnconnected=off
  Mag : Outport  Port=4  VectorParamsAs1DForOutWhenUnconnected=off
  GPS_Lat : Outport  Port=5  VectorParamsAs1DForOutWhenUnconnected=off
  GPS_Lon : Outport  Port=6  VectorParamsAs1DForOutWhenUnconnected=off
  GPS_Alt : Outport  Port=7  VectorParamsAs1DForOutWhenUnconnected=off
  GPS_Speed : Outport  Port=8  VectorParamsAs1DForOutWhenUnconnected=off
  GPS_Course : Outport  Port=9  VectorParamsAs1DForOutWhenUnconnected=off
  GPS_Sats : Outport  Port=10  VectorParamsAs1DForOutWhenUnconnected=off
  GPS_Fix_Age : Outport  Port=11  VectorParamsAs1DForOutWhenUnconnected=off
  wires:
  MATLAB System/3 -> Baro_Alt/1
  MATLAB System1/1 -> RotVel/1
  MATLAB System2/1 -> LinAccel/1
  MATLAB System2/2 -> Mag/1
  MATLAB System3/7 -> GPS_Fix_Age/1
  MATLAB System3/1 -> GPS_Lat/1
  MATLAB System3/2 -> GPS_Lon/1
  MATLAB System3/3 -> GPS_Speed/1
  MATLAB System3/4 -> GPS_Course/1
  MATLAB System3/5 -> GPS_Alt/1
  MATLAB System3/6 -> GPS_Sats/1
  MATLAB System/1 -> Terminator/1
  MATLAB System/2 -> Terminator1/1

== system UAV/Flight Dynamics/Coeff Model/Actuator Aerodynamic Coefficients/Aileron ==
  Actuator : Inport
  Alpha : Inport  Port=2
  Constant1 : Constant  Value=0
  Constant2 : Constant  Value=0
  Constant3 : Constant  Value=0
  Constant4 : Constant  Value=aeroCoeff.Cy_da
  Constant5 : Constant  Value=aeroCoeff.Cl_da_alpha
  Constant6 : Constant  Value=aeroCoeff.Cn_da
  Constant7 : Constant  Value=aeroCoeff.Cl_da
  Mux1 : Mux  Inputs=6
  Product{1..5} (5 alike) : Product  InputSameDT=on  SaturateOnIntegerOverflow=on  OutDataTypeStr=Inherit: Same as first input
  Sum1 : Sum  Inputs=|++
  delCoeff : Outport  VectorParamsAs1DForOutWhenUnconnected=off
  wires:
  Product5/1 -> Sum1/2
  Constant7/1 -> Product5/1
  Sum1/1 -> Mux1/4
  Product4/1 -> Product1/1
  Alpha/1 -> Product4/1
  Constant6/1 -> Product3/2
  Product3/1 -> Mux1/6
  Actuator/1 -> Product2/1, Product3/1, Product5/2, Product4/2
  Product1/1 -> Sum1/1
  Constant5/1 -> Product1/2
  Constant4/1 -> Product2/2
  Constant3/1 -> Mux1/5
  Constant2/1 -> Mux1/3
  Constant1/1 -> Mux1/1
  Mux1/1 -> delCoeff/1
  Product2/1 -> Mux1/2

== system UAV/Flight Dynamics/Coeff Model/Actuator Aerodynamic Coefficients/Elevator ==
  Actuator : Inport
  Beta : Inport  Port=2
  Constant{1..2,4,8} (4 alike) : Constant  Value=0
  Constant5 : Constant  Value=aeroCoeff.Cz_de_beta
  Constant6 : Constant  Value=aeroCoeff.Cm_de
  Constant7 : Constant  Value=aeroCoeff.Cz_de
  Mux1 : Mux  Inputs=6
  Product1 : Product  InputSameDT=on  SaturateOnIntegerOverflow=on  OutDataTypeStr=Inherit: Same as first input
  Product2 : Product  InputSameDT=on  SaturateOnIntegerOverflow=on  OutDataTypeStr=Inherit: Same as first input
  Product3 : Product  InputSameDT=on  SaturateOnIntegerOverflow=on  OutDataTypeStr=Inherit: Same as first input
  Product4 : Product  Inputs=3  InputSameDT=on  SaturateOnIntegerOverflow=on  OutDataTypeStr=Inherit: Same as first input
  Sum : Sum  Inputs=|++
  delCoeff : Outport  VectorParamsAs1DForOutWhenUnconnected=off
  wires:
  Product2/1 -> Sum/2
  Beta/1 -> Product4/1, Product4/2
  Product3/1 -> Mux1/5
  Constant2/1 -> Mux1/6
  Constant8/1 -> Mux1/4
  Constant1/1 -> Mux1/1
  Product1/1 -> Sum/1
  Mux1/1 -> delCoeff/1
  Constant4/1 -> Mux1/2
  Constant7/1 -> Product2/1
  Product4/1 -> Product1/1
  Constant5/1 -> Product1/2
  Constant6/1 -> Product3/2
  Actuator/1 -> Product4/3, Product2/2, Product3/1
  Sum/1 -> Mux1/3

== system UAV/Flight Dynamics/Coeff Model/Actuator Aerodynamic Coefficients/Flap ==
  Actuator : Inport
  Alpha : Inport  Port=2
  Constant1 : Constant  Value=aeroCoeff.Cz_df_alpha
  Constant2 : Constant  Value=aeroCoeff.Cz_df
  Constant3 : Constant  Value=0
  Constant5 : Constant  Value=aeroCoeff.Cx_df_alpha
  Constant6 : Constant  Value=aeroCoeff.Cm_df
  Constant7 : Constant  Value=aeroCoeff.Cx_df
  Constant8 : Constant  Value=0
  Constant9 : Constant  Value=0
  Mux1 : Mux  Inputs=6
  Product{1..7} (7 alike) : Product  InputSameDT=on  SaturateOnIntegerOverflow=on  OutDataTypeStr=Inherit: Same as first input
  Sum2 : Sum  Inputs=++|
  Sum3 : Sum  Inputs=|++
  delCoeff : Outport  VectorParamsAs1DForOutWhenUnconnected=off
  wires:
  Product7/1 -> Sum3/2
  Product6/1 -> Sum2/1
  Product1/1 -> Sum2/2
  Constant1/1 -> Product2/2
  Product5/1 -> Product2/1
  Alpha/1 -> Product5/1, Product4/2
  Constant2/1 -> Product7/1
  Product2/1 -> Sum3/1
  Sum3/1 -> Mux1/3
  Sum2/1 -> Mux1/1
  Product3/1 -> Mux1/5
  Constant9/1 -> Mux1/2
  Constant8/1 -> Mux1/4
  Mux1/1 -> delCoeff/1
  Constant3/1 -> Mux1/6
  Constant7/1 -> Product6/1
  Product4/1 -> Product1/1
  Constant5/1 -> Product1/2
  Constant6/1 -> Product3/2
  Actuator/1 -> Product4/1, Product7/2, Product3/1, Product5/2, Product6/2

== system UAV/Flight Dynamics/Coeff Model/Actuator Aerodynamic Coefficients/Rudder ==
  Actuator : Inport
  Alpha : Inport  Port=2
  Constant1 : Constant  Value=aeroCoeff.Cx_dr
  Constant2 : Constant  Value=0
  Constant3 : Constant  Value=0
  Constant4 : Constant  Value=aeroCoeff.Cl_dr
  Constant5 : Constant  Value=aeroCoeff.Cy_dr_alpha
  Constant6 : Constant  Value=aeroCoeff.Cn_dr
  Constant7 : Constant  Value=aeroCoeff.Cy_dr
  Mux1 : Mux  Inputs=6
  Product{1..6} (6 alike) : Product  InputSameDT=on  SaturateOnIntegerOverflow=on  OutDataTypeStr=Inherit: Same as first input
  Sum1 : Sum  Inputs=|++
  delCoeff : Outport  VectorParamsAs1DForOutWhenUnconnected=off
  wires:
  Product6/1 -> Sum1/2
  Sum1/1 -> Mux1/2
  Product5/1 -> Mux1/1
  Constant1/1 -> Product5/2
  Product2/1 -> Mux1/4
  Product3/1 -> Mux1/6
  Constant4/1 -> Product2/2
  Product1/1 -> Sum1/1
  Mux1/1 -> delCoeff/1
  Constant3/1 -> Mux1/5
  Constant7/1 -> Product6/1
  Constant2/1 -> Mux1/3
  Alpha/1 -> Product4/1
  Product4/1 -> Product1/1
  Constant5/1 -> Product1/2
  Constant6/1 -> Product3/2
  Actuator/1 -> Product5/1, Product4/2, Product6/2, Product2/1, Product3/1

== system UAV/Flight Dynamics/Coeff Model/Aerodynamic Coefficients/Body Rate Damping ==
  V : Inport  Unit=m/s
  Bus Element In : Inport  Port=2  PortName=pqr  Element=p_wind
  Bus Element In1 : Inport  Port=2  PortName=pqr  Element=q_wind
  Bus Element In2 : Inport  Port=2  PortName=pqr  Element=r_wind
  Product : Product  InputSameDT=on  SaturateOnIntegerOverflow=on  OutDataTypeStr=Inherit: Same as first input
  Product1 : Product  InputSameDT=on  SaturateOnIntegerOverflow=on  OutDataTypeStr=Inherit: Same as first input
  Product2 : Product  InputSameDT=on  SaturateOnIntegerOverflow=on  OutDataTypeStr=Inherit: Same as first input
  Product3 : Product  Inputs=*/  InputSameDT=on  SaturateOnIntegerOverflow=on  OutDataTypeStr=Inherit: Same as first input
  Reference Length : Gain  Gain=vehicle.chord  SaturateOnIntegerOverflow=on  OutDataTypeStr=Inherit: Same as input  ParamDataTypeStr=Inherit: Same as input
  Reference Span : Gain  Gain=vehicle.wingspan/2  SaturateOnIntegerOverflow=on  OutDataTypeStr=Inherit: Same as input  ParamDataTypeStr=Inherit: Same as input
  "Reference Span " : Gain  Gain=vehicle.wingspan/2  SaturateOnIntegerOverflow=on  OutDataTypeStr=Inherit: Same as input  ParamDataTypeStr=Inherit: Same as input
  Sum1 : Sum  Inputs=+++  InputSameDT=on  SaturateOnIntegerOverflow=on  OutDataTypeStr=Inherit: Same as first input
  p : Subsystem
  q : Subsystem
  r : Subsystem
  Coeff : Outport  InitialOutput=0  VectorParamsAs1DForOutWhenUnconnected=off
  wires:
  Bus Element In/1 -> Product/2
  Bus Element In1/1 -> Product1/2
  Bus Element In2/1 -> Product2/2
  p/1(delCoeff) -> Product/1
  q/1(delCoeff) -> Product1/1
  Sum1/1 -> Product3/1
  V/1 -> Product3/2
  Product3/1 -> Coeff/1
  Product1/1 -> Reference Length/1
  Product2/1 -> "Reference Span "/1
  Product/1 -> Reference Span/1
  r/1(delCoeff) -> Product2/1
  Reference Length/1 -> Sum1/2
  Reference Span/1 -> Sum1/1
  "Reference Span "/1 -> Sum1/3

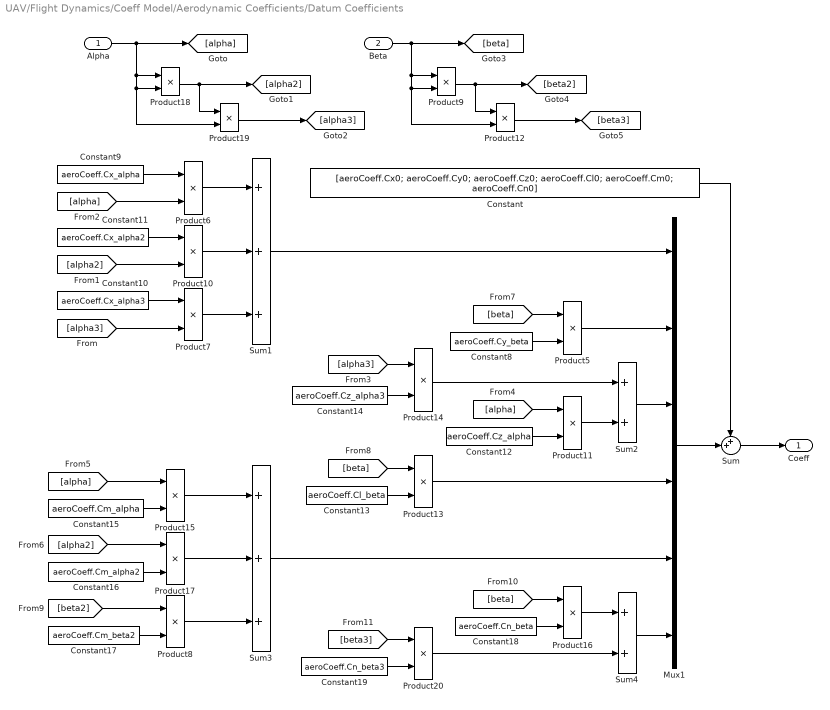
== system UAV/Flight Dynamics/Coeff Model/Aerodynamic Coefficients/Datum Coefficients ==
  Alpha : Inport
  Beta : Inport  Port=2
  Constant : Constant  Value=[aeroCoeff.Cx0; aeroCoeff.Cy0; aeroCoeff.Cz0; aeroCoeff.Cl0; aeroCoeff.Cm0; aeroCoeff.Cn0]
  Constant10 : Constant  Value=aeroCoeff.Cx_alpha3
  Constant11 : Constant  Value=aeroCoeff.Cx_alpha2
  Constant12 : Constant  Value=aeroCoeff.Cz_alpha
  Constant13 : Constant  Value=aeroCoeff.Cl_beta
  Constant14 : Constant  Value=aeroCoeff.Cz_alpha3
  Constant15 : Constant  Value=aeroCoeff.Cm_alpha
  Constant16 : Constant  Value=aeroCoeff.Cm_alpha2
  Constant17 : Constant  Value=aeroCoeff.Cm_beta2
  Constant18 : Constant  Value=aeroCoeff.Cn_beta
  Constant19 : Constant  Value=aeroCoeff.Cn_beta3
  Constant8 : Constant  Value=aeroCoeff.Cy_beta
  Constant9 : Constant  Value=aeroCoeff.Cx_alpha
  Mux1 : Mux  Inputs=6
  Product{5..20} (16 alike) : Product  InputSameDT=on  SaturateOnIntegerOverflow=on  OutDataTypeStr=Inherit: Same as first input
  Sum : Sum  Inputs=++|
  Sum1 : Sum  Inputs=+++  SaturateOnIntegerOverflow=on
  Sum2 : Sum  Inputs=2  SaturateOnIntegerOverflow=on
  Sum3 : Sum  Inputs=+++  SaturateOnIntegerOverflow=on
  Sum4 : Sum  Inputs=2  SaturateOnIntegerOverflow=on
  Coeff : Outport  InitialOutput=0  VectorParamsAs1DForOutWhenUnconnected=off
  wires:
  Sum/1 -> Coeff/1
  Constant/1 -> Sum/1
  Mux1/1 -> Sum/2
  Sum3/1 -> Mux1/5
  Product16/1 -> Sum4/1
  Product20/1 -> Sum4/2
  [beta3] -> Product20/1
  [beta] -> Product16/1
  Constant19/1 -> Product20/2
  Constant18/1 -> Product16/2
  Sum4/1 -> Mux1/6
  [beta2] -> Product8/1
  [beta] -> Product13/1
  [beta] -> Product5/1
  Beta/1 -> Product9/1, Product12/2, Product9/2, [beta]
  Product9/1 -> Product12/1, [beta2]
  Product12/1 -> [beta3]
  Product8/1 -> Sum3/3
  Constant17/1 -> Product8/2
  [alpha] -> Product15/1
  [alpha] -> Product11/1
  [alpha3] -> Product14/1
  [alpha] -> Product6/2
  [alpha2] -> Product10/2
  Constant10/1 -> Product7/1
  [alpha3] -> Product7/2
  Product19/1 -> [alpha3]
  Product18/1 -> [alpha2], Product19/1
  Alpha/1 -> [alpha], Product18/2, Product19/2, Product18/1
  Constant16/1 -> Product17/2
  Product17/1 -> Sum3/2
  [alpha2] -> Product17/1
  Constant15/1 -> Product15/2
  Product15/1 -> Sum3/1
  Constant14/1 -> Product14/2
  Product13/1 -> Mux1/4
  Constant13/1 -> Product13/2
  Sum2/1 -> Mux1/3
  Product14/1 -> Sum2/1
  Product11/1 -> Sum2/2
  Constant12/1 -> Product11/2
  Product10/1 -> Sum1/2
  Product6/1 -> Sum1/1
  Product7/1 -> Sum1/3
  Constant11/1 -> Product10/1
  Constant9/1 -> Product6/1
  Sum1/1 -> Mux1/1
  Product5/1 -> Mux1/2
  Constant8/1 -> Product5/2
